simulink model "simple_streaming_txrx"  (Simulink 6.6)
settings: Solver=ode45  StartTime=0.0  StopTime=inf  RelTol=1e-3
InitFcn:
  | simple_streaming_init
StartFcn:
  | simple_streaming_init
undefined symbols (not defined in the file): dmf, gcbh, get, modConstellation_qam16, modConstellation_qam64, modConstellation_qpsk, rcosfir, symbolRomLen, txLSFR_initValues, txLSFR_polynomials, viqAvgLen, xlBlockLoadCallback, xlGetSimulinkPeriod
libraries: xbsIndex_r4 x506, commchan3 x2, commsink2 x1
(part 5 of 5)

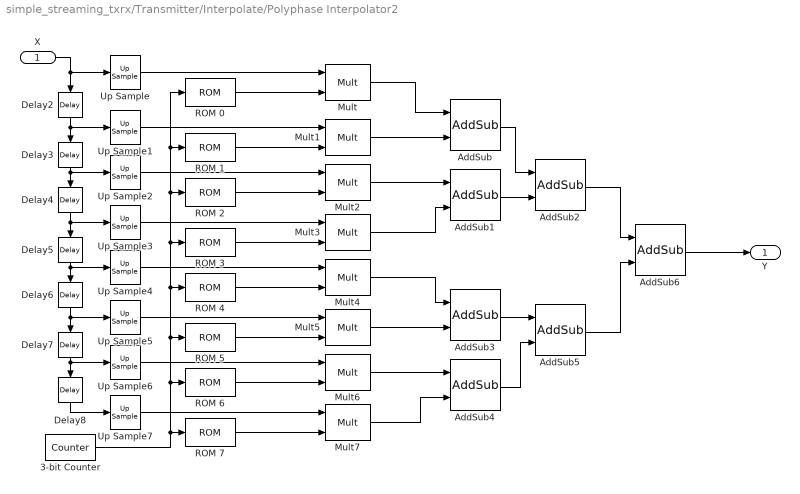
== system simple_streaming_txrx/Transmitter/Interpolate/Polyphase Interpolator2 ==
  X : Inport
  3-bit Counter : xbsIndex_r4/Counter  cnt_type=Free Running  cnt_to=Inf  operation=Up  start_count=1  cnt_by_val=1  arith_type=Unsigned  n_bits=3  bin_pt=0  load_pin=off  rst=off  en=off  explicit_period=off  period=data_samplePeriod / polyphaseBranches  dbl_ovrd=off  use_behavioral_HDL=off  use_rpm=on  block_type=counter
      settings: xl_area=[3 3 0 3 0 0 0]  block_version=10.1
  AddSub{,1,3..4} (4 alike) : xbsIndex_r4/AddSub  mode=Addition  use_carryin=off  use_carryout=off  en=off  latency=0  precision=Full  arith_type=Unsigned  n_bits=8  bin_pt=2  quantization=Truncate  overflow=Wrap  dbl_ovrd=off  use_behavioral_HDL=on  pipelined=off  use_rpm=on  block_type=addsub
      settings: xl_area=[10 0 0 19 0 0 0]  block_version=10.1
  AddSub2 : xbsIndex_r4/AddSub  mode=Addition  use_carryin=off  use_carryout=off  en=off  latency=1  precision=Full  arith_type=Unsigned  n_bits=8  bin_pt=2  quantization=Truncate  overflow=Wrap  dbl_ovrd=off  use_behavioral_HDL=on  pipelined=off  use_rpm=on  block_type=addsub
      settings: xl_area=[11 0 0 20 0 0 0]  block_version=10.1
  AddSub5 : xbsIndex_r4/AddSub  mode=Addition  use_carryin=off  use_carryout=off  en=off  latency=1  precision=Full  arith_type=Unsigned  n_bits=8  bin_pt=2  quantization=Truncate  overflow=Wrap  dbl_ovrd=off  use_behavioral_HDL=on  pipelined=off  use_rpm=on  block_type=addsub
      settings: xl_area=[11 0 0 20 0 0 0]  block_version=10.1
  AddSub6 : xbsIndex_r4/AddSub  mode=Addition  use_carryin=off  use_carryout=off  en=off  latency=0  precision=User Defined  arith_type="Signed  (2's comp)"  n_bits=add_prec  bin_pt=add_bp  quantization=Truncate  overflow=Flag as error  dbl_ovrd=off  use_behavioral_HDL=on  pipelined=off  use_rpm=on  block_type=addsub
      settings: xl_area=[11 0 0 21 0 0 0]  block_version=10.1
  Delay{2..8} (7 alike) : xbsIndex_r4/Delay  Orientation=down  en=off  latency=1  dbl_ovrd=off  reg_retiming=off  block_type=delay
      settings: xl_area=[8 16 0 0 0 0 0]  block_version=10.1
  Mult{,1..7} (8 alike) : xbsIndex_r4/Mult  precision=User Defined  arith_type="Signed  (2's comp)"  n_bits=mult_prec  bin_pt=mult_bp  quantization=Truncate  overflow=Flag as error  en=off  latency=multLatency  dbl_ovrd=off  use_behavioral_HDL=off  use_embedded=on  opt=Speed  optimum_pipeline=off  pipeline=on  use_rpm=on  placement_style=Rectangular shape  block_type=mult
      settings: infoedit=Hardware notes: To use the internal pipeline stage of the dedicated multiplier you must select 'Pipeline for maximum performance'.  xl_area=[9 -11 0 18 0 1 0]  block_version=10.1
  ROM 0 : xbsIndex_r4/ROM  depth=polyphaseBranches  initVector=h(1:subFilterLength)  distributed_mem=Distributed memory  rst=off  init_reg=0  en=off  latency=1  arith_type="Signed  (2's comp)"  n_bits=coeff_prec  bin_pt=coeff_bp  dbl_ovrd=off  optimize=Area  use_rpm=off  block_type=sprom
      settings: xl_area=[7 14 0 14 0 0 0]  block_version=10.1
  ROM 1 : xbsIndex_r4/ROM  depth=polyphaseBranches  initVector=h(1*subFilterLength+1:2*subFilterLength)  distributed_mem=Distributed memory  rst=off  init_reg=0  en=off  latency=1  arith_type="Signed  (2's comp)"  n_bits=coeff_prec  bin_pt=coeff_bp  dbl_ovrd=off  optimize=Area  use_rpm=off  block_type=sprom
      settings: xl_area=[7 14 0 14 0 0 0]  block_version=10.1
  ROM 2 : xbsIndex_r4/ROM  depth=polyphaseBranches  initVector=h(2*subFilterLength+1:3*subFilterLength)  distributed_mem=Distributed memory  rst=off  init_reg=0  en=off  latency=1  arith_type="Signed  (2's comp)"  n_bits=coeff_prec  bin_pt=coeff_bp  dbl_ovrd=off  optimize=Area  use_rpm=off  block_type=sprom
      settings: xl_area=[7 14 0 14 0 0 0]  block_version=10.1
  ROM 3 : xbsIndex_r4/ROM  depth=polyphaseBranches  initVector=h(3*subFilterLength+1:4*subFilterLength)  distributed_mem=Distributed memory  rst=off  init_reg=0  en=off  latency=1  arith_type="Signed  (2's comp)"  n_bits=coeff_prec  bin_pt=coeff_bp  dbl_ovrd=off  optimize=Area  use_rpm=off  block_type=sprom
      settings: xl_area=[7 14 0 14 0 0 0]  block_version=10.1
  ROM 4 : xbsIndex_r4/ROM  depth=polyphaseBranches  initVector=h(4*subFilterLength+1:5*subFilterLength)  distributed_mem=Distributed memory  rst=off  init_reg=0  en=off  latency=1  arith_type="Signed  (2's comp)"  n_bits=coeff_prec  bin_pt=coeff_bp  dbl_ovrd=off  optimize=Area  use_rpm=off  block_type=sprom
      settings: xl_area=[7 14 0 12 0 0 0]  block_version=10.1
  ROM 5 : xbsIndex_r4/ROM  depth=polyphaseBranches  initVector=h(5*subFilterLength+1:6*subFilterLength)  distributed_mem=Distributed memory  rst=off  init_reg=0  en=off  latency=1  arith_type="Signed  (2's comp)"  n_bits=coeff_prec  bin_pt=coeff_bp  dbl_ovrd=off  optimize=Area  use_rpm=off  block_type=sprom
      settings: xl_area=[7 14 0 14 0 0 0]  block_version=10.1
  ROM 6 : xbsIndex_r4/ROM  depth=polyphaseBranches  initVector=h(6*subFilterLength+1:7*subFilterLength)  distributed_mem=Distributed memory  rst=off  init_reg=0  en=off  latency=1  arith_type="Signed  (2's comp)"  n_bits=coeff_prec  bin_pt=coeff_bp  dbl_ovrd=off  optimize=Area  use_rpm=off  block_type=sprom
      settings: xl_area=[7 14 0 14 0 0 0]  block_version=10.1
  ROM 7 : xbsIndex_r4/ROM  depth=polyphaseBranches  initVector=h(7*subFilterLength+1:8*subFilterLength)  distributed_mem=Distributed memory  rst=off  init_reg=0  en=off  latency=1  arith_type="Signed  (2's comp)"  n_bits=coeff_prec  bin_pt=coeff_bp  dbl_ovrd=off  optimize=Area  use_rpm=off  block_type=sprom
      settings: xl_area=[7 14 0 14 0 0 0]  block_version=10.1
  Up Sample{,1..7} (8 alike) : xbsIndex_r4/Up Sample  sample_ratio=polyphaseBranches  copy_samples=on  dbl_ovrd=off  block_type=usamp
      settings: infoedit="Up samples input data.  Inserted values  can be zeros or copies of the most recent input sample.<P><P>Hardware notes: No hardware is needed if inserted values are copies of the input sample; otherwise, a mux and single bit flip-flop are used."  xl_area=[0 0 0 0 0 0 0]  block_version=10.1
  Y : Outport
  wires:
  AddSub6/1 -> Y/1
  Up Sample7/1 -> Mult7/1
  Up Sample6/1 -> Mult6/1
  Up Sample5/1 -> Mult5/1
  Up Sample4/1 -> Mult4/1
  Up Sample3/1 -> Mult3/1
  Up Sample2/1 -> Mult2/1
  Up Sample1/1 -> Mult1/1
  Up Sample/1 -> Mult/1
  AddSub5/1 -> AddSub6/2
  AddSub2/1 -> AddSub6/1
  Mult7/1 -> AddSub4/2
  Mult6/1 -> AddSub4/1
  Mult5/1 -> AddSub3/2
  Mult4/1 -> AddSub3/1
  AddSub4/1 -> AddSub5/2
  AddSub3/1 -> AddSub5/1
  AddSub1/1 -> AddSub2/2
  AddSub/1 -> AddSub2/1
  Mult3/1 -> AddSub1/2
  Mult2/1 -> AddSub1/1
  Mult1/1 -> AddSub/2
  Mult/1 -> AddSub/1
  3-bit Counter/1 -> ROM 7/1, ROM 6/1, ROM 5/1, ROM 4/1, ROM 3/1, ROM 2/1, ROM 1/1, ROM 0/1
  ROM 7/1 -> Mult7/2
  ROM 6/1 -> Mult6/2
  ROM 5/1 -> Mult5/2
  ROM 4/1 -> Mult4/2
  ROM 3/1 -> Mult3/2
  ROM 2/1 -> Mult2/2
  ROM 1/1 -> Mult1/2
  ROM 0/1 -> Mult/2
  X/1 -> Delay2/1, Up Sample/1
  Delay8/1 -> Up Sample7/1
  Delay7/1 -> Up Sample6/1, Delay8/1
  Delay6/1 -> Up Sample5/1, Delay7/1
  Delay5/1 -> Up Sample4/1, Delay6/1
  Delay4/1 -> Up Sample3/1, Delay5/1
  Delay3/1 -> Up Sample2/1, Delay4/1
  Delay2/1 -> Up Sample1/1, Delay3/1

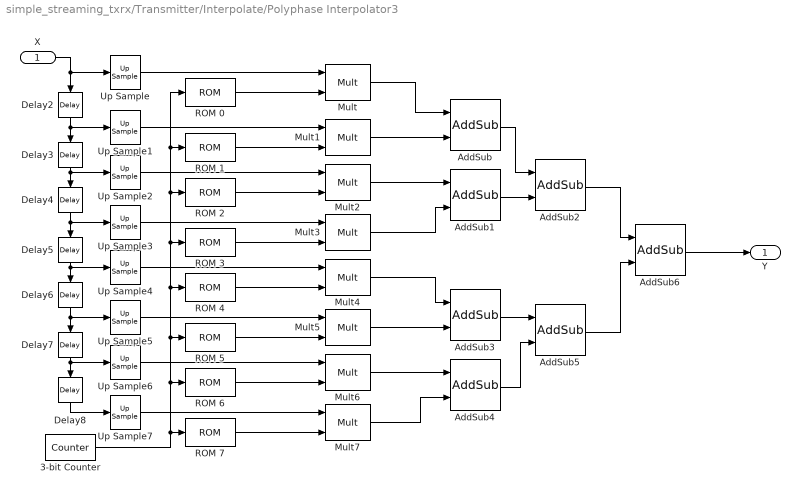
== system simple_streaming_txrx/Transmitter/Interpolate/Polyphase Interpolator3 ==
  X : Inport
  3-bit Counter : xbsIndex_r4/Counter  cnt_type=Free Running  cnt_to=Inf  operation=Up  start_count=1  cnt_by_val=1  arith_type=Unsigned  n_bits=3  bin_pt=0  load_pin=off  rst=off  en=off  explicit_period=off  period=data_samplePeriod / polyphaseBranches  dbl_ovrd=off  use_behavioral_HDL=off  use_rpm=on  block_type=counter
      settings: xl_area=[3 3 0 3 0 0 0]  block_version=10.1
  AddSub{,1,3..4} (4 alike) : xbsIndex_r4/AddSub  mode=Addition  use_carryin=off  use_carryout=off  en=off  latency=0  precision=Full  arith_type=Unsigned  n_bits=8  bin_pt=2  quantization=Truncate  overflow=Wrap  dbl_ovrd=off  use_behavioral_HDL=on  pipelined=off  use_rpm=on  block_type=addsub
      settings: xl_area=[10 0 0 19 0 0 0]  block_version=10.1
  AddSub2 : xbsIndex_r4/AddSub  mode=Addition  use_carryin=off  use_carryout=off  en=off  latency=1  precision=Full  arith_type=Unsigned  n_bits=8  bin_pt=2  quantization=Truncate  overflow=Wrap  dbl_ovrd=off  use_behavioral_HDL=on  pipelined=off  use_rpm=on  block_type=addsub
      settings: xl_area=[11 0 0 20 0 0 0]  block_version=10.1
  AddSub5 : xbsIndex_r4/AddSub  mode=Addition  use_carryin=off  use_carryout=off  en=off  latency=1  precision=Full  arith_type=Unsigned  n_bits=8  bin_pt=2  quantization=Truncate  overflow=Wrap  dbl_ovrd=off  use_behavioral_HDL=on  pipelined=off  use_rpm=on  block_type=addsub
      settings: xl_area=[11 0 0 20 0 0 0]  block_version=10.1
  AddSub6 : xbsIndex_r4/AddSub  mode=Addition  use_carryin=off  use_carryout=off  en=off  latency=0  precision=User Defined  arith_type="Signed  (2's comp)"  n_bits=add_prec  bin_pt=add_bp  quantization=Truncate  overflow=Flag as error  dbl_ovrd=off  use_behavioral_HDL=on  pipelined=off  use_rpm=on  block_type=addsub
      settings: xl_area=[11 0 0 21 0 0 0]  block_version=10.1
  Delay{2..8} (7 alike) : xbsIndex_r4/Delay  Orientation=down  en=off  latency=1  dbl_ovrd=off  reg_retiming=off  block_type=delay
      settings: xl_area=[8 16 0 0 0 0 0]  block_version=10.1
  Mult{,1..7} (8 alike) : xbsIndex_r4/Mult  precision=User Defined  arith_type="Signed  (2's comp)"  n_bits=mult_prec  bin_pt=mult_bp  quantization=Truncate  overflow=Flag as error  en=off  latency=multLatency  dbl_ovrd=off  use_behavioral_HDL=off  use_embedded=on  opt=Speed  optimum_pipeline=off  pipeline=on  use_rpm=on  placement_style=Rectangular shape  block_type=mult
      settings: infoedit=Hardware notes: To use the internal pipeline stage of the dedicated multiplier you must select 'Pipeline for maximum performance'.  xl_area=[9 -11 0 18 0 1 0]  block_version=10.1
  ROM 0 : xbsIndex_r4/ROM  depth=polyphaseBranches  initVector=h(1:subFilterLength)  distributed_mem=Distributed memory  rst=off  init_reg=0  en=off  latency=1  arith_type="Signed  (2's comp)"  n_bits=coeff_prec  bin_pt=coeff_bp  dbl_ovrd=off  optimize=Area  use_rpm=off  block_type=sprom
      settings: xl_area=[7 14 0 14 0 0 0]  block_version=10.1
  ROM 1 : xbsIndex_r4/ROM  depth=polyphaseBranches  initVector=h(1*subFilterLength+1:2*subFilterLength)  distributed_mem=Distributed memory  rst=off  init_reg=0  en=off  latency=1  arith_type="Signed  (2's comp)"  n_bits=coeff_prec  bin_pt=coeff_bp  dbl_ovrd=off  optimize=Area  use_rpm=off  block_type=sprom
      settings: xl_area=[7 14 0 14 0 0 0]  block_version=10.1
  ROM 2 : xbsIndex_r4/ROM  depth=polyphaseBranches  initVector=h(2*subFilterLength+1:3*subFilterLength)  distributed_mem=Distributed memory  rst=off  init_reg=0  en=off  latency=1  arith_type="Signed  (2's comp)"  n_bits=coeff_prec  bin_pt=coeff_bp  dbl_ovrd=off  optimize=Area  use_rpm=off  block_type=sprom
      settings: xl_area=[7 14 0 14 0 0 0]  block_version=10.1
  ROM 3 : xbsIndex_r4/ROM  depth=polyphaseBranches  initVector=h(3*subFilterLength+1:4*subFilterLength)  distributed_mem=Distributed memory  rst=off  init_reg=0  en=off  latency=1  arith_type="Signed  (2's comp)"  n_bits=coeff_prec  bin_pt=coeff_bp  dbl_ovrd=off  optimize=Area  use_rpm=off  block_type=sprom
      settings: xl_area=[7 14 0 14 0 0 0]  block_version=10.1
  ROM 4 : xbsIndex_r4/ROM  depth=polyphaseBranches  initVector=h(4*subFilterLength+1:5*subFilterLength)  distributed_mem=Distributed memory  rst=off  init_reg=0  en=off  latency=1  arith_type="Signed  (2's comp)"  n_bits=coeff_prec  bin_pt=coeff_bp  dbl_ovrd=off  optimize=Area  use_rpm=off  block_type=sprom
      settings: xl_area=[7 14 0 12 0 0 0]  block_version=10.1
  ROM 5 : xbsIndex_r4/ROM  depth=polyphaseBranches  initVector=h(5*subFilterLength+1:6*subFilterLength)  distributed_mem=Distributed memory  rst=off  init_reg=0  en=off  latency=1  arith_type="Signed  (2's comp)"  n_bits=coeff_prec  bin_pt=coeff_bp  dbl_ovrd=off  optimize=Area  use_rpm=off  block_type=sprom
      settings: xl_area=[7 14 0 14 0 0 0]  block_version=10.1
  ROM 6 : xbsIndex_r4/ROM  depth=polyphaseBranches  initVector=h(6*subFilterLength+1:7*subFilterLength)  distributed_mem=Distributed memory  rst=off  init_reg=0  en=off  latency=1  arith_type="Signed  (2's comp)"  n_bits=coeff_prec  bin_pt=coeff_bp  dbl_ovrd=off  optimize=Area  use_rpm=off  block_type=sprom
      settings: xl_area=[7 14 0 14 0 0 0]  block_version=10.1
  ROM 7 : xbsIndex_r4/ROM  depth=polyphaseBranches  initVector=h(7*subFilterLength+1:8*subFilterLength)  distributed_mem=Distributed memory  rst=off  init_reg=0  en=off  latency=1  arith_type="Signed  (2's comp)"  n_bits=coeff_prec  bin_pt=coeff_bp  dbl_ovrd=off  optimize=Area  use_rpm=off  block_type=sprom
      settings: xl_area=[7 14 0 14 0 0 0]  block_version=10.1
  Up Sample{,1..7} (8 alike) : xbsIndex_r4/Up Sample  sample_ratio=polyphaseBranches  copy_samples=on  dbl_ovrd=off  block_type=usamp
      settings: infoedit="Up samples input data.  Inserted values  can be zeros or copies of the most recent input sample.<P><P>Hardware notes: No hardware is needed if inserted values are copies of the input sample; otherwise, a mux and single bit flip-flop are used."  xl_area=[0 0 0 0 0 0 0]  block_version=10.1
  Y : Outport
  wires:
  Delay2/1 -> Delay3/1, Up Sample1/1
  Delay3/1 -> Delay4/1, Up Sample2/1
  Delay4/1 -> Delay5/1, Up Sample3/1
  Delay5/1 -> Delay6/1, Up Sample4/1
  Delay6/1 -> Delay7/1, Up Sample5/1
  Delay7/1 -> Delay8/1, Up Sample6/1
  Delay8/1 -> Up Sample7/1
  X/1 -> Up Sample/1, Delay2/1
  ROM 0/1 -> Mult/2
  ROM 1/1 -> Mult1/2
  ROM 2/1 -> Mult2/2
  ROM 3/1 -> Mult3/2
  ROM 4/1 -> Mult4/2
  ROM 5/1 -> Mult5/2
  ROM 6/1 -> Mult6/2
  ROM 7/1 -> Mult7/2
  3-bit Counter/1 -> ROM 0/1, ROM 1/1, ROM 2/1, ROM 3/1, ROM 4/1, ROM 5/1, ROM 6/1, ROM 7/1
  Mult/1 -> AddSub/1
  Mult1/1 -> AddSub/2
  Mult2/1 -> AddSub1/1
  Mult3/1 -> AddSub1/2
  AddSub/1 -> AddSub2/1
  AddSub1/1 -> AddSub2/2
  AddSub3/1 -> AddSub5/1
  AddSub4/1 -> AddSub5/2
  Mult4/1 -> AddSub3/1
  Mult5/1 -> AddSub3/2
  Mult6/1 -> AddSub4/1
  Mult7/1 -> AddSub4/2
  AddSub2/1 -> AddSub6/1
  AddSub5/1 -> AddSub6/2
  Up Sample/1 -> Mult/1
  Up Sample1/1 -> Mult1/1
  Up Sample2/1 -> Mult2/1
  Up Sample3/1 -> Mult3/1
  Up Sample4/1 -> Mult4/1
  Up Sample5/1 -> Mult5/1
  Up Sample6/1 -> Mult6/1
  Up Sample7/1 -> Mult7/1
  AddSub6/1 -> Y/1

== system simple_streaming_txrx/Transmitter/Random Symbols/6bit Datasource ==
  Concat{1..4} (4 alike) : xbsIndex_r4/Concat  num_inputs=2  dbl_ovrd=off  block_type=concat
      settings: block_version=10.1
  LFSR : xbsIndex_r4/LFSR  lfsr_type=Fibonacci  gate_type=XOR  n_bits=txLSFR_numBits  polynomial=txLSFR_polynomials{1}  rst_value=txLSFR_initValues{1}  rst=off  en=off  reloadable_seed=off  input_type=off  output_type=off  arith_type=Unsigned  bin_pt=4  dbl_ovrd=off  explicit_period=on  period=1  block_type=lfsr
      settings: xl_area=[0, 0, 0, 0, 0, 0, 0]  block_version=10.1
  LFSR1 : xbsIndex_r4/LFSR  lfsr_type=Fibonacci  gate_type=XOR  n_bits=txLSFR_numBits  polynomial=txLSFR_polynomials{2}  rst_value=txLSFR_initValues{2}  rst=off  en=off  reloadable_seed=off  input_type=off  output_type=off  arith_type=Unsigned  bin_pt=4  dbl_ovrd=off  explicit_period=on  period=1  block_type=lfsr
      settings: xl_area=[0, 0, 0, 0, 0, 0, 0]  block_version=10.1
  LFSR2 : xbsIndex_r4/LFSR  lfsr_type=Fibonacci  gate_type=XOR  n_bits=txLSFR_numBits  polynomial=txLSFR_polynomials{3}  rst_value=txLSFR_initValues{3}  rst=off  en=off  reloadable_seed=off  input_type=off  output_type=off  arith_type=Unsigned  bin_pt=4  dbl_ovrd=off  explicit_period=on  period=1  block_type=lfsr
      settings: xl_area=[0, 0, 0, 0, 0, 0, 0]  block_version=10.1
  LFSR3 : xbsIndex_r4/LFSR  lfsr_type=Fibonacci  gate_type=XOR  n_bits=txLSFR_numBits  polynomial=txLSFR_polynomials{4}  rst_value=txLSFR_initValues{4}  rst=off  en=off  reloadable_seed=off  input_type=off  output_type=off  arith_type=Unsigned  bin_pt=4  dbl_ovrd=off  explicit_period=on  period=1  block_type=lfsr
      settings: xl_area=[0, 0, 0, 0, 0, 0, 0]  block_version=10.1
  LFSR4 : xbsIndex_r4/LFSR  lfsr_type=Fibonacci  gate_type=XOR  n_bits=txLSFR_numBits  polynomial=txLSFR_polynomials{5}  rst_value=txLSFR_initValues{5}  rst=off  en=off  reloadable_seed=off  input_type=off  output_type=off  arith_type=Unsigned  bin_pt=4  dbl_ovrd=off  explicit_period=on  period=1  block_type=lfsr
      settings: xl_area=[0, 0, 0, 0, 0, 0, 0]  block_version=10.1
  LFSR5 : xbsIndex_r4/LFSR  lfsr_type=Fibonacci  gate_type=XOR  n_bits=txLSFR_numBits  polynomial=txLSFR_polynomials{6}  rst_value=txLSFR_initValues{6}  rst=off  en=off  reloadable_seed=off  input_type=off  output_type=off  arith_type=Unsigned  bin_pt=4  dbl_ovrd=off  explicit_period=on  period=1  block_type=lfsr
      settings: xl_area=[0, 0, 0, 0, 0, 0, 0]  block_version=10.1
  I : Outport
  Q : Outport  Port=2
  wires:
  LFSR/1 -> Concat1/1
  LFSR1/1 -> Concat1/2
  Concat1/1 -> Concat2/1
  LFSR2/1 -> Concat2/2
  Concat3/1 -> Concat4/1
  LFSR5/1 -> Concat4/2
  LFSR3/1 -> Concat3/1
  LFSR4/1 -> Concat3/2
  Concat2/1 -> I/1
  Concat4/1 -> Q/1

== system simple_streaming_txrx/Transmitter/Random Symbols/Modulation ==
  Mod Sel : Inport
  I Bits : Inport  Port=2
  Q Bits : Inport  Port=3
  16QAM Mapper : xbsIndex_r4/ROM  depth=length(modConstellation_qam16)  initVector=modConstellation_qam16./max(abs(modConstellation_qam16))  distributed_mem=Distributed memory  rst=off  init_reg=0  en=off  latency=1  arith_type="Signed  (2's comp)"  n_bits=8  bin_pt=7  dbl_ovrd=off  optimize=Area  use_rpm=off  block_type=sprom
      settings: xl_area=[4 8 0 8 0 0 0]  block_version=10.1
  16QAM Mapper1 : xbsIndex_r4/ROM  depth=length(modConstellation_qam16)  initVector=modConstellation_qam16  distributed_mem=Distributed memory  rst=off  init_reg=0  en=off  latency=1  arith_type="Signed  (2's comp)"  n_bits=8  bin_pt=7  dbl_ovrd=off  optimize=Area  use_rpm=off  block_type=sprom
      settings: xl_area=[4 8 0 8 0 0 0]  block_version=10.1
  2LSB : xbsIndex_r4/Slice  nbits=2  boolean_output=off  mode=Lower Bit Location + Width  bit1=0  base1=MSB of Input  bit0=0  base0=LSB of Input  dbl_ovrd=off  block_type=slice
      settings: infoedit="Extracts a given range of bits from each input sample and presents it at the output.  The output type is ordinarily unsigned with binary point at zero, but can be Boolean when the slice is one bit wide.<P><P>Hardware notes: In hardware this block costs nothing."  block_version=10.1
  2LSB1 : xbsIndex_r4/Slice  nbits=2  boolean_output=off  mode=Lower Bit Location + Width  bit1=0  base1=MSB of Input  bit0=0  base0=LSB of Input  dbl_ovrd=off  block_type=slice
      settings: infoedit="Extracts a given range of bits from each input sample and presents it at the output.  The output type is ordinarily unsigned with binary point at zero, but can be Boolean when the slice is one bit wide.<P><P>Hardware notes: In hardware this block costs nothing."  block_version=10.1
  64QAM Mapper : xbsIndex_r4/ROM  depth=length(modConstellation_qam64)  initVector=modConstellation_qam64  distributed_mem=Distributed memory  rst=off  init_reg=0  en=off  latency=1  arith_type="Signed  (2's comp)"  n_bits=8  bin_pt=7  dbl_ovrd=off  optimize=Area  use_rpm=off  block_type=sprom
      settings: xl_area=[4 8 0 8 0 0 0]  block_version=10.1
  64QAM Mapper1 : xbsIndex_r4/ROM  depth=length(modConstellation_qam64)  initVector=modConstellation_qam64  distributed_mem=Block RAM  rst=off  init_reg=0  en=off  latency=1  arith_type="Signed  (2's comp)"  n_bits=8  bin_pt=7  dbl_ovrd=off  optimize=Area  use_rpm=off  block_type=sprom
      settings: xl_area=[0 0 1 0 0 0 0]  block_version=10.1
  Constant7 : xbsIndex_r4/Constant  arith_type=Signed (2's comp)  const=0  n_bits=8  bin_pt=7  explicit_period=on  period=1  equ=P=C  opselect=C  inp2=PCIN>>17  opr=+  inp1=P  carry=CIN  dbl_ovrd=off  block_type=constant
      settings: block_version=10.1
  Counter : xbsIndex_r4/Counter  cnt_type=Free Running  cnt_to=Inf  operation=Up  start_count=0  cnt_by_val=1  arith_type=Unsigned  n_bits=log2(symbolRomLen)  bin_pt=0  load_pin=off  rst=off  en=off  explicit_period=on  period=1  dbl_ovrd=off  use_behavioral_HDL=off  use_rpm=off  block_type=counter
      settings: xl_area=[8 13 0 13 0 0 0]  block_version=10.1
  LSB : xbsIndex_r4/Slice  nbits=1  boolean_output=off  mode=Lower Bit Location + Width  bit1=0  base1=MSB of Input  bit0=0  base0=LSB of Input  dbl_ovrd=off  block_type=slice
      settings: infoedit="Extracts a given range of bits from each input sample and presents it at the output.  The output type is ordinarily unsigned with binary point at zero, but can be Boolean when the slice is one bit wide.<P><P>Hardware notes: In hardware this block costs nothing."  block_version=10.1
  MSB : xbsIndex_r4/Slice  nbits=1  boolean_output=off  mode=Lower Bit Location + Width  bit1=0  base1=MSB of Input  bit0=0  base0=MSB of Input  dbl_ovrd=off  block_type=slice
      settings: infoedit="Extracts a given range of bits from each input sample and presents it at the output.  The output type is ordinarily unsigned with binary point at zero, but can be Boolean when the slice is one bit wide.<P><P>Hardware notes: In hardware this block costs nothing."  block_version=10.1
  Mux2 : xbsIndex_r4/Mux  inputs=4  en=off  latency=1  precision=Full  arith_type="Signed  (2's comp)"  n_bits=8  bin_pt=2  quantization=Truncate  overflow=Wrap  dbl_ovrd=off  block_type=mux
      settings: xl_area=[8 8 0 16 0 0 0]  block_version=10.1
  Mux3 : xbsIndex_r4/Mux  inputs=4  en=off  latency=1  precision=Full  arith_type="Signed  (2's comp)"  n_bits=8  bin_pt=2  quantization=Truncate  overflow=Wrap  dbl_ovrd=off  block_type=mux
      settings: xl_area=[8 8 0 16 0 0 0]  block_version=10.1
  QPSK Map : Subsystem
  QPSK Map1 : Subsystem
  ROM : xbsIndex_r4/ROM  depth=symbolRomLen  initVector=symbolRom  distributed_mem=Block RAM  rst=off  init_reg=0  en=off  latency=1  arith_type=Unsigned  n_bits=2  bin_pt=0  dbl_ovrd=off  optimize=Area  use_rpm=on  block_type=sprom
      settings: xl_area=[0 0 1 0 0 0 0]  block_version=10.1
  I : Outport
  Q : Outport  Port=2
  wires:
  64QAM Mapper1/1 -> Mux3/5
  16QAM Mapper1/1 -> Mux3/4
  Constant7/1 -> Mux3/2, Mux2/2
  QPSK Map1/1(Sym) -> Mux3/3
  64QAM Mapper/1 -> Mux2/5
  16QAM Mapper/1 -> Mux2/4
  QPSK Map/1(Sym) -> Mux2/3
  Mod Sel/1 -> Mux3/1, Mux2/1
  2LSB1/1 -> 16QAM Mapper1/1
  2LSB/1 -> 16QAM Mapper/1
  I Bits/1 -> 64QAM Mapper/1, 2LSB/1
  Mux2/1 -> I/1
  Mux3/1 -> Q/1
  Q Bits/1 -> 64QAM Mapper1/1, 2LSB1/1
  ROM/1 -> LSB/1, MSB/1
  LSB/1 -> QPSK Map/1(Bit)
  MSB/1 -> QPSK Map1/1(Bit)
  Counter/1 -> ROM/1

== system simple_streaming_txrx/Transmitter/Upconverter/ComplexMult ==
  A I : Inport
  A Q : Inport  Port=2
  B I : Inport  Port=3
  B Q : Inport  Port=4
  AddSub : xbsIndex_r4/AddSub  mode=Subtraction  use_carryin=off  use_carryout=off  en=off  latency=0  precision=User Defined  arith_type="Signed  (2's comp)"  n_bits=16  bin_pt=15  quantization=Truncate  overflow=Wrap  dbl_ovrd=off  use_behavioral_HDL=off  pipelined=off  use_rpm=on  block_type=addsub
      settings: xl_area=[8 0 0 16 0 0 0]  block_version=10.1
  AddSub1 : xbsIndex_r4/AddSub  mode=Addition  use_carryin=off  use_carryout=off  en=off  latency=0  precision=User Defined  arith_type="Signed  (2's comp)"  n_bits=16  bin_pt=15  quantization=Truncate  overflow=Wrap  dbl_ovrd=off  use_behavioral_HDL=off  pipelined=off  use_rpm=on  block_type=addsub
      settings: xl_area=[8 0 0 16 0 0 0]  block_version=10.1
  Convert : xbsIndex_r4/Convert  arith_type="Signed  (2's comp)"  n_bits=16  bin_pt=15  quantization=Truncate  overflow=Wrap  latency=0  dbl_ovrd=off  pipeline=off  block_type=convert
      settings: xl_area=[0 0 0 0 0 0 0]  block_version=10.1
  Convert1 : xbsIndex_r4/Convert  arith_type="Signed  (2's comp)"  n_bits=16  bin_pt=15  quantization=Truncate  overflow=Wrap  latency=0  dbl_ovrd=off  pipeline=off  block_type=convert
      settings: xl_area=[0 0 0 0 0 0 0]  block_version=10.1
  Mult{,1..3} (4 alike) : xbsIndex_r4/Mult  precision=User Defined  arith_type="Signed  (2's comp)"  n_bits=16  bin_pt=15  quantization=Truncate  overflow=Wrap  en=off  latency=1  dbl_ovrd=off  use_behavioral_HDL=off  use_embedded=on  opt=Speed  optimum_pipeline=off  pipeline=on  use_rpm=on  placement_style=Triangular  block_type=mult
      settings: infoedit=Hardware notes: To use the internal pipeline stage of the dedicated multiplier you must select 'Pipeline for maximum performance'.  xl_area=[8 -15 0 16 0 1 0]  block_version=10.1
  Scale : xbsIndex_r4/Scale  scale_factor=-1  dbl_ovrd=off  block_type=scale
      settings: infoedit=Scales input by a power of two by adjusting the binary point position.<P><P>Hardware notes: In hardware this block costs nothing.  block_version=10.1
  Scale1 : xbsIndex_r4/Scale  scale_factor=-1  dbl_ovrd=off  block_type=scale
      settings: infoedit=Scales input by a power of two by adjusting the binary point position.<P><P>Hardware notes: In hardware this block costs nothing.  block_version=10.1
  I : Outport
  Q : Outport  Port=2
  wires:
  Mult/1 -> AddSub/1
  Mult1/1 -> AddSub/2
  Mult2/1 -> AddSub1/1
  Mult3/1 -> AddSub1/2
  AddSub/1 -> Scale/1
  AddSub1/1 -> Scale1/1
  Scale/1 -> Convert/1
  Scale1/1 -> Convert1/1
  A I/1 -> Mult/1, Mult3/1
  B I/1 -> Mult/2, Mult2/2
  A Q/1 -> Mult1/1, Mult2/1
  B Q/1 -> Mult1/2, Mult3/2
  Convert/1 -> I/1
  Convert1/1 -> Q/1

== system simple_streaming_txrx/Transmitter/Upconverter/Re[A*B] ==
  A I : Inport
  A Q : Inport  Port=2
  B I : Inport  Port=3
  B Q : Inport  Port=4
  Gateway Out1 : xbsIndex_r4/Gateway Out  hdl_port=off  timing_constraint=None  locs_specified=off  LOCs={}  block_type=gatewayout
      settings: infoedit="Gateway out block.  Converts Xilinx fixed point inputs into ouputs of type Simulink integer, double, or fixed point.<P><P>Hardware notes:  In hardware these blocks become top level output ports or are discarded, depending on how they are configured."  xl_area=[0 0 0 0 0 0 0]  block_version=10.1
  Gateway Out5 : xbsIndex_r4/Gateway Out  hdl_port=off  timing_constraint=None  locs_specified=off  LOCs={}  block_type=gatewayout
      settings: infoedit="Gateway out block.  Converts Xilinx fixed point inputs into ouputs of type Simulink integer, double, or fixed point.<P><P>Hardware notes:  In hardware these blocks become top level output ports or are discarded, depending on how they are configured."  xl_area=[0 0 0 0 0 0 0]  block_version=10.1
  Scale : xbsIndex_r4/Scale  scale_factor=-1  dbl_ovrd=off  block_type=scale
      settings: infoedit=Scales input by a power of two by adjusting the binary point position.<P><P>Hardware notes: In hardware this block costs nothing.  block_version=10.1
  To Workspace : ToWorkspace  VariableName=Symbols_I  SampleTime=-1  SaveFormat=Array
  To Workspace1 : ToWorkspace  VariableName=Carrier_I  SampleTime=-1  SaveFormat=Array
  i1i2 : xbsIndex_r4/Mult  precision=User Defined  arith_type="Signed  (2's comp)"  n_bits=14  bin_pt=13  quantization=Truncate  overflow=Saturate  en=off  latency=1  dbl_ovrd=off  use_behavioral_HDL=off  use_embedded=on  opt=Speed  optimum_pipeline=off  pipeline=on  use_rpm=on  placement_style=Rectangular shape  block_type=mult
      settings: infoedit=Hardware notes: To use the internal pipeline stage of the dedicated multiplier you must select 'Pipeline for maximum performance'.  xl_area=[15 -17 0 29 0 1 0]  block_version=10.1
  i1i2 plus q1q2 : xbsIndex_r4/AddSub  mode=Subtraction  use_carryin=off  use_carryout=off  en=off  latency=0  precision=User Defined  arith_type="Signed  (2's comp)"  n_bits=14  bin_pt=12  quantization=Truncate  overflow=Flag as error  dbl_ovrd=off  use_behavioral_HDL=on  pipelined=off  use_rpm=on  block_type=addsub
      settings: xl_area=[8 0 0 15 0 0 0]  block_version=10.1
  i1i4 : xbsIndex_r4/Mult  precision=User Defined  arith_type="Signed  (2's comp)"  n_bits=14  bin_pt=13  quantization=Truncate  overflow=Saturate  en=off  latency=1  dbl_ovrd=off  use_behavioral_HDL=off  use_embedded=on  opt=Speed  optimum_pipeline=off  pipeline=on  use_rpm=on  placement_style=Rectangular shape  block_type=mult
      settings: infoedit=Hardware notes: To use the internal pipeline stage of the dedicated multiplier you must select 'Pipeline for maximum performance'.  xl_area=[15 -17 0 29 0 1 0]  block_version=10.1
  Out : Outport
  wires:
  i1i4/1 -> i1i2 plus q1q2/2
  i1i2/1 -> i1i2 plus q1q2/1
  B Q/1 -> i1i4/2
  A Q/1 -> i1i4/1
  B I/1 -> i1i2/2, Gateway Out1/1
  A I/1 -> i1i2/1, Gateway Out5/1
  i1i2 plus q1q2/1 -> Scale/1
  Scale/1 -> Out/1
  Gateway Out5/1 -> To Workspace/1
  Gateway Out1/1 -> To Workspace1/1

== system simple_streaming_txrx/Transmitter/Upconverter/myDDS ==
  phase inc : Inport
  10MSB : xbsIndex_r4/Slice  nbits=10  boolean_output=off  mode=Upper Bit Location + Width  bit1=0  base1=MSB of Input  bit0=0  base0=LSB of Input  dbl_ovrd=off  block_type=slice
      settings: infoedit="Extracts a given range of bits from each input sample and presents it at the output.  The output type is ordinarily unsigned with binary point at zero, but can be Boolean when the slice is one bit wide.<P><P>Hardware notes: In hardware this block costs nothing."  block_version=10.1
  Accumulator : xbsIndex_r4/Accumulator  operation=Add  n_bits=32  overflow=Wrap  scale=1  rst=off  hasbypass=off  en=off  dbl_ovrd=off  use_behavioral_HDL=on  block_type=accum
      settings: infoedit="Adder or subtractor-based accumulator.   Output type and binary point position match the input.<P><P>Hardware notes: When \"Reinitialize with input 'b' on reset\" is selected, the accumulator is forced to run at the system rate even if the input 'b' is running at a slower rate."  xl_area=[16 32 0 32 0 0 0]  block_version=10.1
  Cos ROM : xbsIndex_r4/ROM  depth=1024  initVector=cos(2*pi*[0:1023]/1024)  distributed_mem=Block RAM  rst=off  init_reg=0  en=off  latency=1  arith_type="Signed  (2's comp)"  n_bits=16  bin_pt=15  dbl_ovrd=off  optimize=Area  use_rpm=off  block_type=sprom
      settings: xl_area=[0 0 1 0 0 0 0]  block_version=10.1
  Sin ROM : xbsIndex_r4/ROM  depth=1024  initVector=sin(2*pi*[0:1023]/1024)  distributed_mem=Block RAM  rst=off  init_reg=0  en=off  latency=1  arith_type="Signed  (2's comp)"  n_bits=16  bin_pt=15  dbl_ovrd=off  optimize=Area  use_rpm=off  block_type=sprom
      settings: xl_area=[0 0 1 0 0 0 0]  block_version=10.1
  sin : Outport
  cos : Outport  Port=2
  wires:
  Accumulator/1 -> 10MSB/1
  phase inc/1 -> Accumulator/1
  Cos ROM/1 -> cos/1
  Sin ROM/1 -> sin/1
  10MSB/1 -> Cos ROM/1, Sin ROM/1

== system simple_streaming_txrx/Receiver/AGC Hook/Fine/Subsystem ==
  S : Inport
  R : Inport  Port=2
  Constant1 : xbsIndex_r4/Constant  arith_type=Boolean  const=1  n_bits=1  bin_pt=0  explicit_period=off  period=1  equ=P=C  opselect=C  inp2=PCIN>>17  opr=+  inp1=P  carry=CIN  dbl_ovrd=off  block_type=constant
      settings: block_version=10.1.2
  Register : xbsIndex_r4/Register  init=0  rst=on  en=on  dbl_ovrd=off  block_type=register
      settings: block_version=10.1.2
  O : Outport
  wires:
  Constant1/1 -> Register/1
  S/1 -> Register/3
  R/1 -> Register/2
  Register/1 -> O/1

== system simple_streaming_txrx/Receiver/AGC Hook/Fine/posedge ==
  In1 : Inport
  Delay : xbsIndex_r4/Delay  en=off  latency=1  dbl_ovrd=off  reg_retiming=off  block_type=delay
      settings: block_version=10.1.2
  Inverter : xbsIndex_r4/Inverter  en=off  latency=0  dbl_ovrd=off  block_type=inv
      settings: block_version=10.1.2
  Logical : xbsIndex_r4/Logical  logical_function=AND  inputs=2  en=off  latency=0  precision=Full  arith_type=Unsigned  n_bits=16  bin_pt=0  align_bp=on  dbl_ovrd=off  block_type=logical
      settings: block_version=10.1.2
  Out1 : Outport
  wires:
  In1/1 -> Delay/1, Logical/1
  Delay/1 -> Inverter/1
  Inverter/1 -> Logical/2
  Logical/1 -> Out1/1

== system simple_streaming_txrx/Receiver/Decimate & Filter/I MF1/Adder Tree ==
  In1 : Inport
  In2 : Inport  Port=2
  In3 : Inport  Port=3
  In4 : Inport  Port=4
  In5 : Inport  Port=5
  In6 : Inport  Port=6
  In7 : Inport  Port=7
  In8 : Inport  Port=8
  AddSub{,1,3..4} (4 alike) : xbsIndex_r4/AddSub  mode=Addition  use_carryin=off  use_carryout=off  en=off  latency=0  precision=Full  arith_type=Unsigned  n_bits=8  bin_pt=2  quantization=Truncate  overflow=Wrap  dbl_ovrd=off  use_behavioral_HDL=on  pipelined=off  use_rpm=on  block_type=addsub
      settings: xl_area=[10 0 0 19 0 0 0]  block_version=10.1
  AddSub2 : xbsIndex_r4/AddSub  mode=Addition  use_carryin=off  use_carryout=off  en=off  latency=1  precision=Full  arith_type=Unsigned  n_bits=8  bin_pt=2  quantization=Truncate  overflow=Wrap  dbl_ovrd=off  use_behavioral_HDL=on  pipelined=off  use_rpm=on  block_type=addsub
      settings: xl_area=[11 0 0 20 0 0 0]  block_version=10.1
  AddSub5 : xbsIndex_r4/AddSub  mode=Addition  use_carryin=off  use_carryout=off  en=off  latency=1  precision=Full  arith_type=Unsigned  n_bits=8  bin_pt=2  quantization=Truncate  overflow=Wrap  dbl_ovrd=off  use_behavioral_HDL=on  pipelined=off  use_rpm=on  block_type=addsub
      settings: xl_area=[11 0 0 20 0 0 0]  block_version=10.1
  AddSub6 : xbsIndex_r4/AddSub  mode=Addition  use_carryin=off  use_carryout=off  en=off  latency=0  precision=User Defined  arith_type="Signed  (2's comp)"  n_bits=add_prec  bin_pt=add_bp  quantization=Truncate  overflow=Flag as error  dbl_ovrd=off  use_behavioral_HDL=on  pipelined=off  use_rpm=on  block_type=addsub
      settings: xl_area=[11 0 0 21 0 0 0]  block_version=10.1
  Out1 : Outport
  wires:
  AddSub5/1 -> AddSub6/2
  AddSub2/1 -> AddSub6/1
  AddSub4/1 -> AddSub5/2
  AddSub3/1 -> AddSub5/1
  AddSub1/1 -> AddSub2/2
  AddSub/1 -> AddSub2/1
  In1/1 -> AddSub/1
  In2/1 -> AddSub/2
  In3/1 -> AddSub1/1
  In4/1 -> AddSub1/2
  AddSub6/1 -> Out1/1
  In5/1 -> AddSub3/1
  In6/1 -> AddSub3/2
  In7/1 -> AddSub4/1
  In8/1 -> AddSub4/2

== system simple_streaming_txrx/Receiver/Decimate & Filter/I MF2/Adder Tree ==
  In1 : Inport
  In2 : Inport  Port=2
  In3 : Inport  Port=3
  In4 : Inport  Port=4
  In5 : Inport  Port=5
  In6 : Inport  Port=6
  In7 : Inport  Port=7
  In8 : Inport  Port=8
  AddSub{,1,3..4} (4 alike) : xbsIndex_r4/AddSub  mode=Addition  use_carryin=off  use_carryout=off  en=off  latency=0  precision=Full  arith_type=Unsigned  n_bits=8  bin_pt=2  quantization=Truncate  overflow=Wrap  dbl_ovrd=off  use_behavioral_HDL=on  pipelined=off  use_rpm=on  block_type=addsub
      settings: xl_area=[10 0 0 19 0 0 0]  block_version=10.1
  AddSub2 : xbsIndex_r4/AddSub  mode=Addition  use_carryin=off  use_carryout=off  en=off  latency=1  precision=Full  arith_type=Unsigned  n_bits=8  bin_pt=2  quantization=Truncate  overflow=Wrap  dbl_ovrd=off  use_behavioral_HDL=on  pipelined=off  use_rpm=on  block_type=addsub
      settings: xl_area=[11 0 0 20 0 0 0]  block_version=10.1
  AddSub5 : xbsIndex_r4/AddSub  mode=Addition  use_carryin=off  use_carryout=off  en=off  latency=1  precision=Full  arith_type=Unsigned  n_bits=8  bin_pt=2  quantization=Truncate  overflow=Wrap  dbl_ovrd=off  use_behavioral_HDL=on  pipelined=off  use_rpm=on  block_type=addsub
      settings: xl_area=[11 0 0 20 0 0 0]  block_version=10.1
  AddSub6 : xbsIndex_r4/AddSub  mode=Addition  use_carryin=off  use_carryout=off  en=off  latency=0  precision=User Defined  arith_type="Signed  (2's comp)"  n_bits=add_prec  bin_pt=add_bp  quantization=Truncate  overflow=Flag as error  dbl_ovrd=off  use_behavioral_HDL=on  pipelined=off  use_rpm=on  block_type=addsub
      settings: xl_area=[11 0 0 21 0 0 0]  block_version=10.1
  Out1 : Outport
  wires:
  In8/1 -> AddSub4/2
  In7/1 -> AddSub4/1
  In6/1 -> AddSub3/2
  In5/1 -> AddSub3/1
  AddSub6/1 -> Out1/1
  In4/1 -> AddSub1/2
  In3/1 -> AddSub1/1
  In2/1 -> AddSub/2
  In1/1 -> AddSub/1
  AddSub/1 -> AddSub2/1
  AddSub1/1 -> AddSub2/2
  AddSub3/1 -> AddSub5/1
  AddSub4/1 -> AddSub5/2
  AddSub2/1 -> AddSub6/1
  AddSub5/1 -> AddSub6/2

== system simple_streaming_txrx/Receiver/Decimate & Filter/dMF/Adder Tree ==
  In1 : Inport
  In2 : Inport  Port=2
  In3 : Inport  Port=3
  In4 : Inport  Port=4
  In5 : Inport  Port=5
  In6 : Inport  Port=6
  In7 : Inport  Port=7
  In8 : Inport  Port=8
  AddSub{,1,3..4} (4 alike) : xbsIndex_r4/AddSub  mode=Addition  use_carryin=off  use_carryout=off  en=off  latency=0  precision=Full  arith_type=Unsigned  n_bits=8  bin_pt=2  quantization=Truncate  overflow=Wrap  dbl_ovrd=off  use_behavioral_HDL=on  pipelined=off  use_rpm=on  block_type=addsub
      settings: xl_area=[10 0 0 19 0 0 0]  block_version=10.1
  AddSub2 : xbsIndex_r4/AddSub  mode=Addition  use_carryin=off  use_carryout=off  en=off  latency=1  precision=Full  arith_type=Unsigned  n_bits=8  bin_pt=2  quantization=Truncate  overflow=Wrap  dbl_ovrd=off  use_behavioral_HDL=on  pipelined=off  use_rpm=on  block_type=addsub
      settings: xl_area=[11 0 0 20 0 0 0]  block_version=10.1
  AddSub5 : xbsIndex_r4/AddSub  mode=Addition  use_carryin=off  use_carryout=off  en=off  latency=1  precision=Full  arith_type=Unsigned  n_bits=8  bin_pt=2  quantization=Truncate  overflow=Wrap  dbl_ovrd=off  use_behavioral_HDL=on  pipelined=off  use_rpm=on  block_type=addsub
      settings: xl_area=[11 0 0 20 0 0 0]  block_version=10.1
  AddSub6 : xbsIndex_r4/AddSub  mode=Addition  use_carryin=off  use_carryout=off  en=off  latency=0  precision=User Defined  arith_type="Signed  (2's comp)"  n_bits=add_prec  bin_pt=add_bp  quantization=Truncate  overflow=Flag as error  dbl_ovrd=off  use_behavioral_HDL=on  pipelined=off  use_rpm=on  block_type=addsub
      settings: xl_area=[11 0 0 21 0 0 0]  block_version=10.1
  Out1 : Outport
  wires:
  AddSub5/1 -> AddSub6/2
  AddSub2/1 -> AddSub6/1
  AddSub4/1 -> AddSub5/2
  AddSub3/1 -> AddSub5/1
  AddSub1/1 -> AddSub2/2
  AddSub/1 -> AddSub2/1
  In1/1 -> AddSub/1
  In2/1 -> AddSub/2
  In3/1 -> AddSub1/1
  In4/1 -> AddSub1/2
  AddSub6/1 -> Out1/1
  In5/1 -> AddSub3/1
  In6/1 -> AddSub3/2
  In7/1 -> AddSub4/1
  In8/1 -> AddSub4/2

== system simple_streaming_txrx/Transmitter/Random Symbols/Modulation/QPSK Map ==
  Bit : Inport
  Constant6 : xbsIndex_r4/Constant  arith_type=Signed (2's comp)  const=modConstellation_qpsk(1)  n_bits=8  bin_pt=7  explicit_period=on  period=1  equ=P=C  opselect=C  inp2=PCIN>>17  opr=+  inp1=P  carry=CIN  dbl_ovrd=off  block_type=constant
      settings: block_version=10.1
  Constant7 : xbsIndex_r4/Constant  arith_type=Signed (2's comp)  const=modConstellation_qpsk(2)  n_bits=8  bin_pt=7  explicit_period=on  period=1  equ=P=C  opselect=C  inp2=PCIN>>17  opr=+  inp1=P  carry=CIN  dbl_ovrd=off  block_type=constant
      settings: block_version=10.1
  Mux2 : xbsIndex_r4/Mux  inputs=2  en=off  latency=1  precision=Full  arith_type="Signed  (2's comp)"  n_bits=8  bin_pt=2  quantization=Truncate  overflow=Wrap  dbl_ovrd=off  block_type=mux
      settings: xl_area=[4 8 0 8 0 0 0]  block_version=10.1
  Sym : Outport
  wires:
  Constant6/1 -> Mux2/2
  Constant7/1 -> Mux2/3
  Bit/1 -> Mux2/1
  Mux2/1 -> Sym/1

== system simple_streaming_txrx/Transmitter/Random Symbols/Modulation/QPSK Map1 ==
  Bit : Inport
  Constant6 : xbsIndex_r4/Constant  arith_type=Signed (2's comp)  const=modConstellation_qpsk(1)  n_bits=8  bin_pt=7  explicit_period=on  period=1  equ=P=C  opselect=C  inp2=PCIN>>17  opr=+  inp1=P  carry=CIN  dbl_ovrd=off  block_type=constant
      settings: block_version=10.1
  Constant7 : xbsIndex_r4/Constant  arith_type=Signed (2's comp)  const=modConstellation_qpsk(2)  n_bits=8  bin_pt=7  explicit_period=on  period=1  equ=P=C  opselect=C  inp2=PCIN>>17  opr=+  inp1=P  carry=CIN  dbl_ovrd=off  block_type=constant
      settings: block_version=10.1
  Mux2 : xbsIndex_r4/Mux  inputs=2  en=off  latency=1  precision=Full  arith_type="Signed  (2's comp)"  n_bits=8  bin_pt=2  quantization=Truncate  overflow=Wrap  dbl_ovrd=off  block_type=mux
      settings: xl_area=[4 8 0 8 0 0 0]  block_version=10.1
  Sym : Outport
  wires:
  Mux2/1 -> Sym/1
  Bit/1 -> Mux2/1
  Constant7/1 -> Mux2/3
  Constant6/1 -> Mux2/2
